simulink model "Pi_Noise_Test"  (R2025b)
settings: Solver=FixedStepDiscrete  StartTime=0.0  StopTime=tspan  FixedStep=dt_control  RelTol=1e-3
values from neighbouring files (symbols this model uses):
  mask = obj.total_mask + mask    [maneuver_old.m]
undefined symbols (not defined in the file or in its folder): dt_control, start, stop, Tmax
settings Model: Creator=vulcangrip  LastModifiedBy=kjhaydon
settings OptimizationCC: DefaultParameterBehavior=Inlined  EnhancedBackFolding=on  PassReuseOutputArgsAs=Individual arguments  ZeroExternalMemoryAtStartup=off  ZeroInternalMemoryAtStartup=off  MaxStackSize=64  OptimizeBlockOrder=speed  DifferentSizesBufferReuse=on  OptimizationCustomize=off  EfficientTunableParamExpr=on
settings DebuggingCC: ParameterTunabilityLossMsg=error
settings HardwareCC: ProdBitPerLong=64.0  ProdHWDeviceType=Intel->x86-64 (Linux 64)
settings SFSimCC: MATLABDynamicMemAlloc=off  SimTargetLang=C++  SimDLTargetLibrary=mkl-dnn
settings RTWCC: SystemTargetFile=ert.tlc  HardwareBoard=Robot Operating System 2 (ROS 2)  TLCOptions="-aInlineSetEventsForThisBaseRateFcn=TLC_FALSE -aSuppressMultiTaskScheduler=TLC_FALSE  -aRateBasedStepFcn=0"  GenCodeOnly=on  TemplateMakefile=ert_default_tmf  Toolchain=Colcon Tools  TargetLang=C++  CheckMdlBeforeBuild=Warning  Description=Embedded Coder
settings CodeAppCC: ForceParamTrailComments=on  IgnoreCustomStorageClasses=off  OperatorAnnotations=on  SimulinkDataObjDesc=on  SFDataObjDesc=on  InsertBlockDesc=on
settings ERTTargetCC: ExtModeTransport=2.0  ExtModeStaticAlloc=on  ExtModeAutomaticAllocSize=off  ExtModeMexFile=ext_xcp  ExtModeIntrfLevel=Level2 - Open  RootIOFormat=Structure reference  TargetLangStandard=C++11 (ISO)  CodeInterfacePackaging=C++ class  SubcomponentCodeInterfacePackaging=C++ class

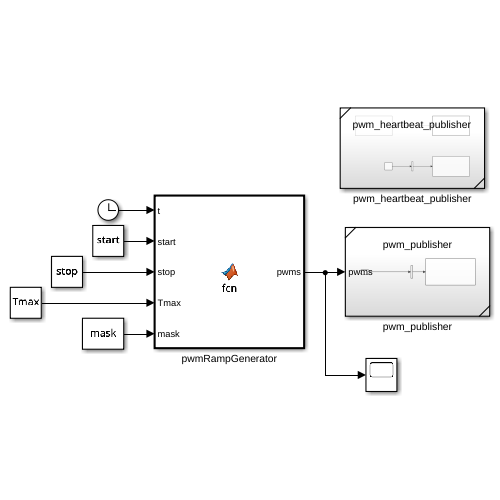
[thumbnail: Simulink's stored preview of the top-level diagram]
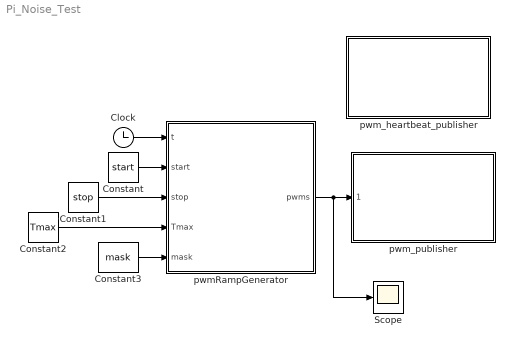
== system Pi_Noise_Test ==
  Clock : Clock
  Constant : Constant  Value=start
  Constant1 : Constant  Value=stop
  Constant2 : Constant  Value=Tmax
  Constant3 : Constant  Value=mask
  Scope : Scope
      settings: ActiveDisplayYMinimum=1475  ActiveDisplayYMaximum=1725
  pwmRampGenerator : MATLAB Function  TreatAsAtomicUnit=on  SystemSampleTime=dt_control
  pwm_heartbeat_publisher : Subsystem  ReferencedSubsystem=pwm_heartbeat_publisher
  pwm_publisher : Subsystem  ReferencedSubsystem=pwm_publisher
  wires:
  Clock/1 -> pwmRampGenerator/1(t)
  pwmRampGenerator/1(pwms) -> Scope/1, pwm_publisher/1
  Constant/1 -> pwmRampGenerator/2(start)
  Constant1/1 -> pwmRampGenerator/3(stop)
  Constant2/1 -> pwmRampGenerator/4(Tmax)
  Constant3/1 -> pwmRampGenerator/5(mask)

== matlab function Pi_Noise_Test/pwmRampGenerator ==
  data: t input; pwms output; start input; stop input; Tmax input; mask input
function pwms = fcn(t, start, stop, Tmax, mask)

pwms = pwmRampGenerator(t, start, stop, Tmax, mask);
